simulink model "Carsimenv"  (R2023b)
settings: Solver=VariableStepAuto  StartTime=0.0  StopTime=150  FixedStep=0.1  RelTol=1e-3  EnableMultiTasking=on
libraries: Solver_SF x1
settings Model: Creator=xuwei  LastModifiedBy=shown
settings SolverCC: AlgebraicLoopSolver=TrustRegion
settings DataIOCC: LimitDataPoints=on  SaveFormat=Array  SignalLoggingSaveFormat=ModelDataLogs  ReturnWorkspaceOutputs=off
settings OptimizationCC: ReuseModelBlockBuffer=off  ExpressionDepthLimit=2147483647  LifeSpan=inf
settings DebuggingCC: UnderspecifiedInitializationDetection=Classic  MergeDetectMultiDrivingBlocksExec=none  SolverPrmCheckMsg=warning  FcnCallInpInsideContextMsg=warning  UnconnectedInputMsg=warning  UnconnectedOutputMsg=warning  UnconnectedLineMsg=warning  StateNameClashWarn=warning  SFUnexpectedBacktrackingDiag=warning  SFNoUnconditionalDefaultTransitionDiag=warning  SFExecutionAtInitializationDiag=none  ArithmeticOperatorsInVariantConditions=warning
settings HardwareCC: ProdBitPerPointer=32  ProdBitPerSizeT=32  ProdBitPerPtrDiffT=32  ProdLargestAtomicFloat=None  ProdIntDivRoundTo=Undefined  ProdEndianess=Unspecified  ProdWordSize=32  ProdHWDeviceType=32-bit Generic
settings ModelReferenceCC: PropagateSignalLabelsOutOfModel=off
settings SFSimCC: SimUseLocalCustomCode=off  CustomCodeUndefinedFunction=UseInterfaceOnly
settings RTWCC: RTWUseLocalCustomCode=off  DLArmComputeVersion=19.05
settings CodeAppCC: StateflowObjectComments=on
settings GRTTargetCC: TargetLangStandard=C89/C90 (ANSI)  CombineOutputUpdateFcns=off  GRTInterface=on
settings ConfigComp: CovMetricSettings=dw  CovSaveCumulativeToWorkspaceVar=on  CovSaveSingleToWorkspaceVar=on  CovExternalEMLEnable=off
settings SimscapeCC: SimscapeNormalizeSystem=off
settings ConfigurationSet: Description=SimMechanics 2G

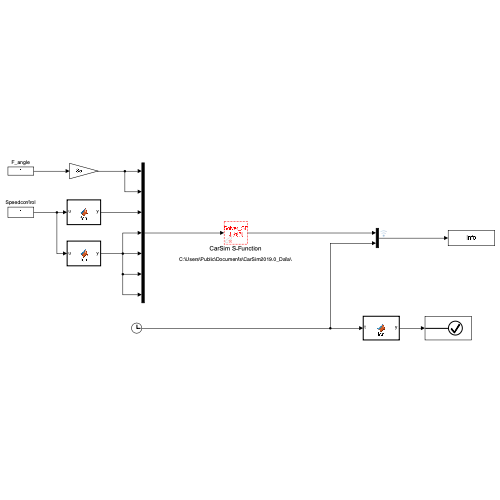
[thumbnail: Simulink's stored preview of the top-level diagram]
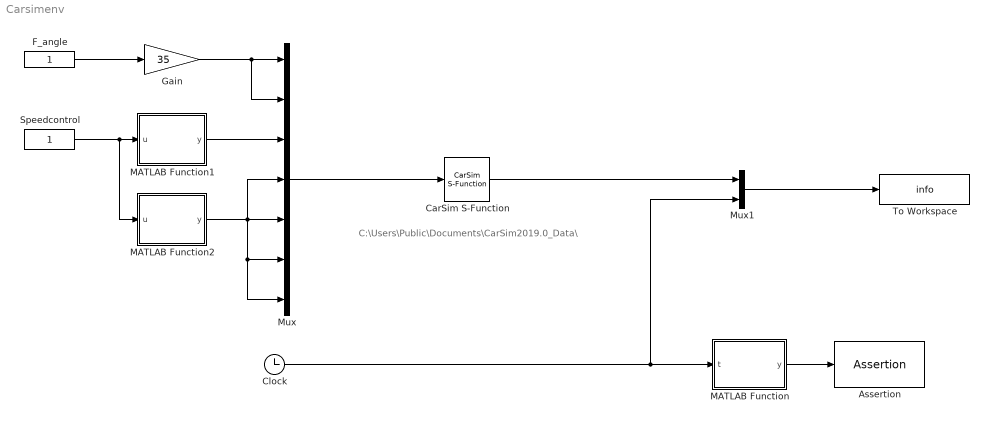
== system Carsimenv ==
  note: C:\Users\Public\Documents\CarSim2019.0_Data\
  Assertion : Assertion  AssertionFailFcn=set_param('Carsimenv','SimulationCommand','pause');  StopWhenAssertionFail=off
  CarSim S-Function : Solver_SF/CarSim S-Function  Priority=1  SIMFILE=C:\Users\Public\Documents\CarSim2019.0_Data\simfile.sim
  Clock : Clock
  F_angle : Constant
  Gain : Gain  Gain=35
  MATLAB Function : MATLAB Function  TreatAsAtomicUnit=on
  MATLAB Function1 : MATLAB Function  TreatAsAtomicUnit=on
  MATLAB Function2 : MATLAB Function  TreatAsAtomicUnit=on
  Mux : Mux  Inputs=7
  Mux1 : Mux  Inputs=2
  Speedcontrol : Constant
  To Workspace : ToWorkspace  VariableName=info  SampleTime=-1
  wires:
  Mux/1 -> CarSim S-Function/1
  F_angle/1 -> Gain/1
  CarSim S-Function/1 -> Mux1/1
  Clock/1 -> Mux1/2, MATLAB Function/1(t)
  MATLAB Function/1(y) -> Assertion/1
  Mux1/1 -> To Workspace/1
  Gain/1 -> Mux/1, Mux/2
  MATLAB Function1/1(y) -> Mux/3
  MATLAB Function2/1(y) -> Mux/7, Mux/6, Mux/5, Mux/4
  Speedcontrol/1 -> MATLAB Function2/1(u), MATLAB Function1/1(u)

== matlab function Carsimenv/MATLAB Function ==
  data: t input; y output
function y = fcn(t)
if  t == 0
    y = 1;
elseif mod(t,0.1) == 0
    y = 0;
else
    y = 1;
end

== matlab function Carsimenv/MATLAB Function2 ==
  data: u input; y output
function y = fcn(u)
if u >= 0
    y = 0;
else
    y = 12*u;
end

== matlab function Carsimenv/MATLAB Function1 ==
  data: u input; y output
function y = fcn(u)
if u >= 0
    y = u;
else
    y = 0;
end
